simulink model "otimizadorpid"  (Simulink 4.00)
settings: Solver=ode45  StartTime=0.0  StopTime=100  RelTol=1e-3
values from neighbouring files (symbols this model uses):
  kd = 0    [ncd1.m]    (also in otimizador.mat; otimizadorpid.mat; sistemacomotimizador.mat)
  ki = 0    [ncd1.m]    (also in otimizador.mat = 7.92912218826; otimizadorpid.mat = 1.40132847448e-08; sistemacomotimizador.mat = 9.74275715262)
  kp = 10    [ncd1.m]    (also in otimizador.mat = 61.1189520833; otimizadorpid.mat = 9.99999996763; sistemacomotimizador.mat = 54.6230709883)
libraries: simulink3 x3
settings Model: LastModifiedBy=Gui  LimitDataPoints=off  ExtModeTrigMode=oneshot  ExtModeArmWhenConnect=off

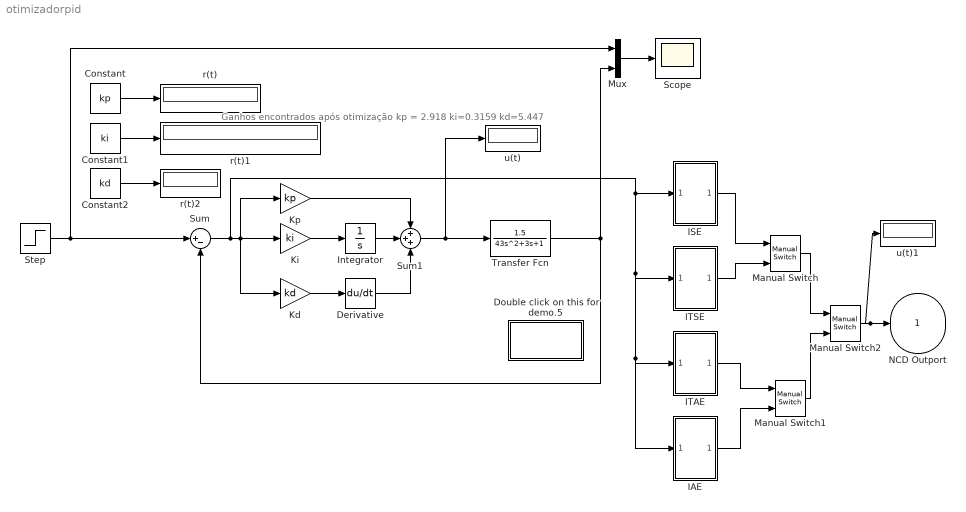
== system otimizadorpid ==
  note: Ganhos encontrados
      | após otimização
      | kp = 2.918
      | ki=0.3159
      | kd=5.447
  Constant : Constant  Value=kp
  Constant1 : Constant  Value=ki
  Constant2 : Constant  Value=kd
  Derivative : Derivative
  Double click on this for demo.5 : Subsystem
      settings: OpenFcn=ncd1  RTWFcnNameOpts=Auto  RTWFileNameOpts=Auto
      mask Display: disp('ncd1')
  IAE : Subsystem
      settings: RTWFcnNameOpts=Auto  RTWFileNameOpts=Auto
  ISE : Subsystem
      settings: RTWFcnNameOpts=Auto  RTWFileNameOpts=Auto
  ITAE : Subsystem
      settings: RTWFcnNameOpts=Auto  RTWFileNameOpts=Auto
  ITSE : Subsystem
      settings: RTWFcnNameOpts=Auto  RTWFileNameOpts=Auto
  Integrator : Integrator  ExternalReset=none  InitialConditionSource=internal  InitialCondition=0  LimitOutput=off  UpperSaturationLimit=inf  LowerSaturationLimit=-inf  ShowSaturationPort=off  ShowStatePort=off  AbsoluteTolerance=auto
  Kd : Gain  Gain=kd  Multiplication=Element-wise(K.*u)  SaturateOnIntegerOverflow=on
  Ki : Gain  Gain=ki  Multiplication=Element-wise(K.*u)  SaturateOnIntegerOverflow=on
  Kp : Gain  Gain=kp  Multiplication=Element-wise(K.*u)  SaturateOnIntegerOverflow=on
  Manual Switch : simulink3/Nonlinear/Manual Switch  sw=1  action=0
  Manual Switch1 : simulink3/Nonlinear/Manual Switch  sw=0  action=0
  Manual Switch2 : simulink3/Nonlinear/Manual Switch  sw=0  action=0
  Mux : Mux  Inputs=2
  Scope : Scope
      settings: TickLabels=on  TimeRange=100  YMin=0.993  YMax=1  SaveToWorkspace=off  SaveName=ScopeData  LimitDataPoints=on  MaxDataPoints=5000
  Step : Step  Time=0.1  Before=0  After=1  SampleTime=0
  Sum : Sum  Inputs=|+-  SaturateOnIntegerOverflow=on
  Sum1 : Sum  Inputs=+++  SaturateOnIntegerOverflow=on
  Transfer Fcn : TransferFcn  Numerator=[1.5]  Denominator=[43 3 1]  AbsoluteTolerance=auto  Realization=auto
  r(t) : Display
      settings: Format=short
  r(t)1 : Display
      settings: Format=short
  r(t)2 : Display
      settings: Format=short
  u(t) : Display
      settings: Format=short
  u(t)1 : Display
      settings: Format=short
  NCD Outport : Outport  Port=1  InitialOutput=0
      settings: OpenFcn=optblock
      mask Type: NCD Outport
      mask Display:
      | plot([0:10],[-.5 1.5 .6 1.3 .8 1.1 .95 1.02 .99 1 1]);
      | disp('\n\n NCD\n OutPort 1');
  wires:
  Step/1 -> Mux/1, Sum/1
  Mux/1 -> Scope/1
  Constant2/1 -> r(t)2/1
  Constant/1 -> r(t)/1
  Constant1/1 -> r(t)1/1
  Transfer Fcn/1 -> Mux/2, Sum/2
  Ki/1 -> Integrator/1
  Kd/1 -> Derivative/1
  Sum/1 -> Ki/1, Kp/1, Kd/1, ISE/1(In1), ITSE/1(In1), ITAE/1(In1), IAE/1(In1)
  Kp/1 -> Sum1/1
  Integrator/1 -> Sum1/2
  Sum1/1 -> Transfer Fcn/1, u(t)/1
  Derivative/1 -> Sum1/3
  ISE/1(Out1) -> Manual Switch/1
  ITSE/1(Out1) -> Manual Switch/2
  ITAE/1(Out1) -> Manual Switch1/1
  IAE/1(Out1) -> Manual Switch1/2
  Manual Switch/1 -> Manual Switch2/1
  Manual Switch1/1 -> Manual Switch2/2
  Manual Switch2/1 -> NCD Outport/1, u(t)1/1

== system otimizadorpid/Double click on this for demo.5 ==

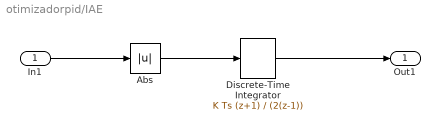
== system otimizadorpid/IAE ==
  In1 : Inport  Port=1  LatchInput=off
  Abs : Abs  SaturateOnIntegerOverflow=on
  Discrete-Time Integrator : DiscreteIntegrator  IntegratorMethod=Trapezoidal  ExternalReset=none  InitialConditionSource=internal  InitialCondition=0  LimitOutput=off  UpperSaturationLimit=inf  LowerSaturationLimit=-inf  ShowSaturationPort=off  ShowStatePort=off  SampleTime=0.1
      settings: RTWStateStorageClass=Auto
  Out1 : Outport  Port=1
  wires:
  Abs/1 -> Discrete-Time Integrator/1
  In1/1 -> Abs/1
  Discrete-Time Integrator/1 -> Out1/1

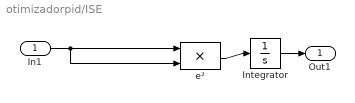
== system otimizadorpid/ISE ==
  In1 : Inport  Port=1  LatchInput=off  SampleTime=1
  Integrator : Integrator  ExternalReset=none  InitialConditionSource=internal  InitialCondition=0  LimitOutput=off  UpperSaturationLimit=inf  LowerSaturationLimit=-inf  ShowSaturationPort=off  ShowStatePort=off  AbsoluteTolerance=auto
  e² : Product  Inputs=2  Multiplication=Element-wise(.*)  SaturateOnIntegerOverflow=on
  Out1 : Outport  Port=1
  wires:
  e²/1 -> Integrator/1
  In1/1 -> e²/1, e²/2
  Integrator/1 -> Out1/1

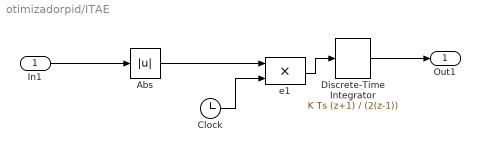
== system otimizadorpid/ITAE ==
  In1 : Inport  Port=1  LatchInput=off
  Abs : Abs  SaturateOnIntegerOverflow=on
  Clock : Clock
      settings: DisplayTime=off  Decimation=10
  Discrete-Time Integrator : DiscreteIntegrator  IntegratorMethod=Trapezoidal  ExternalReset=none  InitialConditionSource=internal  InitialCondition=0  LimitOutput=off  UpperSaturationLimit=inf  LowerSaturationLimit=-inf  ShowSaturationPort=off  ShowStatePort=off  SampleTime=0.1
      settings: RTWStateStorageClass=Auto
  e1 : Product  Inputs=2  Multiplication=Element-wise(.*)  SaturateOnIntegerOverflow=on
  Out1 : Outport  Port=1
  wires:
  Abs/1 -> e1/1
  e1/1 -> Discrete-Time Integrator/1
  Clock/1 -> e1/2
  In1/1 -> Abs/1
  Discrete-Time Integrator/1 -> Out1/1

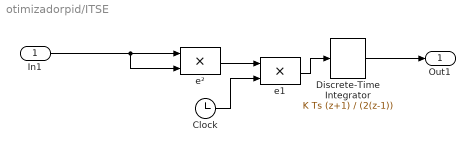
== system otimizadorpid/ITSE ==
  In1 : Inport  Port=1  LatchInput=off
  Clock : Clock
      settings: DisplayTime=off  Decimation=10
  Discrete-Time Integrator : DiscreteIntegrator  IntegratorMethod=Trapezoidal  ExternalReset=none  InitialConditionSource=internal  InitialCondition=0  LimitOutput=off  UpperSaturationLimit=inf  LowerSaturationLimit=-inf  ShowSaturationPort=off  ShowStatePort=off  SampleTime=0.1
      settings: RTWStateStorageClass=Auto
  e1 : Product  Inputs=2  Multiplication=Element-wise(.*)  SaturateOnIntegerOverflow=on
  e² : Product  Inputs=2  Multiplication=Element-wise(.*)  SaturateOnIntegerOverflow=on
  Out1 : Outport  Port=1
  wires:
  In1/1 -> e²/1, e²/2
  e²/1 -> e1/1
  e1/1 -> Discrete-Time Integrator/1
  Clock/1 -> e1/2
  Discrete-Time Integrator/1 -> Out1/1
